simulink subsystem "Aerodyn"  (R2023b)
settings: Solver=VariableStepAuto  StartTime=0.0  StopTime=10.0  RelTol=1e-3
undefined symbols (not defined in the file): Aerodynamics
settings Model: Creator=NicolasS  LastModifiedBy=rouve
settings SolverCC: AlgebraicLoopSolver=TrustRegion
settings DebuggingCC: UnconnectedInputMsg=warning  UnconnectedOutputMsg=warning  UnconnectedLineMsg=warning
settings ModelReferenceCC: EnableRefExpFcnMdlSchedulingChecks=on
settings RTWCC: DLArmComputeVersion=19.05

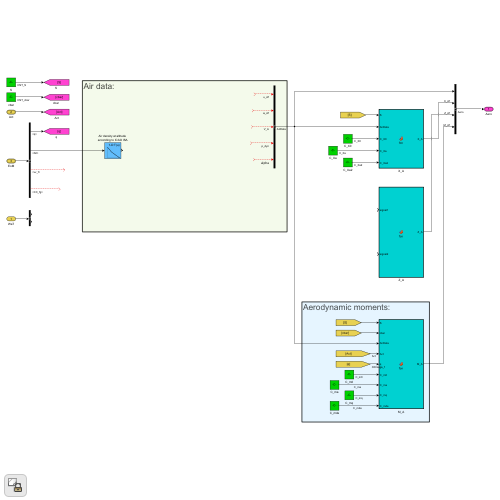
[thumbnail: Simulink's stored preview of the top-level diagram]
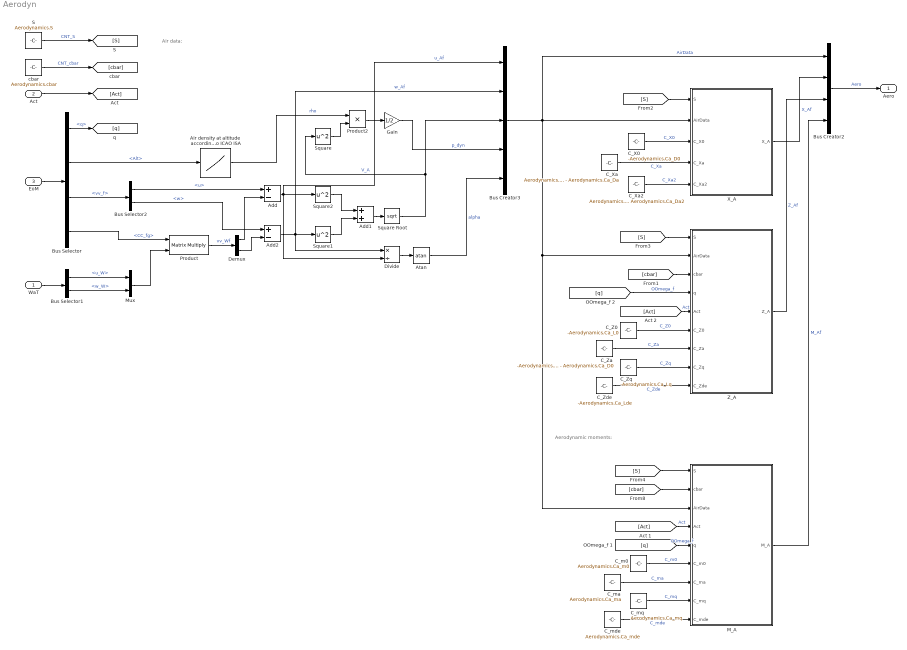
== system Aerodyn ==
  note: Aerodynamic moments:
  note: Air data:
  WaT : Inport  OutDataTypeStr=Bus: WaT
  Act : Inport  Port=2  OutDataTypeStr=Bus: Act
  EoM : Inport  Port=3  OutDataTypeStr=Bus: EoM
  Add : Sum  Inputs=+-
  Add1 : Sum
  Add2 : Sum  Inputs=+-
  Air density at altitude according to ICAO ISA : Lookup_n-D  NumberOfTableDimensions=1  BreakpointsForDimension1=Aerodynamics.LUT_Alt  Table=Aerodynamics.LUT_rho  ExtrapMethod=Clip  InternalRulePriority=Speed  RndMeth=Simplest
  Atan : Trigonometry  Operator=atan
  Bus Creator2 : BusCreator  Inputs=4  OutDataTypeStr=Bus: Aero
  Bus Creator3 : BusCreator  Inputs=5  OutDataTypeStr=Bus: AirData
  Bus Selector : BusSelector  OutputSignals=q,Alt,vv_f,CC.CC_fg
  Bus Selector1 : BusSelector  OutputSignals=u_W,w_W
  Bus Selector2 : BusSelector  OutputSignals=u,w
  C_X0 : Constant  Value=-Aerodynamics.Ca_D0  VectorParams1D=off  OutDataTypeStr=double  SampleTime=-1
  C_Xa : Constant  Value=Aerodynamics.Ca_L0 - Aerodynamics.Ca_Da  VectorParams1D=off  OutDataTypeStr=double  SampleTime=-1
  C_Xa2 : Constant  Value=Aerodynamics.Ca_La - Aerodynamics.Ca_Da2  VectorParams1D=off  OutDataTypeStr=double  SampleTime=-1
  C_Z0 : Constant  Value=-Aerodynamics.Ca_L0  VectorParams1D=off  OutDataTypeStr=double  SampleTime=-1
  C_Za : Constant  Value=-Aerodynamics.Ca_La - Aerodynamics.Ca_D0  VectorParams1D=off  OutDataTypeStr=double  SampleTime=-1
  C_Zde : Constant  Value=-Aerodynamics.Ca_Lde  VectorParams1D=off  OutDataTypeStr=double  SampleTime=-1
  C_Zq : Constant  Value=-Aerodynamics.Ca_Lq  VectorParams1D=off  OutDataTypeStr=double  SampleTime=-1
  C_m0 : Constant  Value=Aerodynamics.Ca_m0  VectorParams1D=off  OutDataTypeStr=double  SampleTime=-1
  C_ma : Constant  Value=Aerodynamics.Ca_ma  VectorParams1D=off  OutDataTypeStr=double  SampleTime=-1
  C_mde : Constant  Value=Aerodynamics.Ca_mde  VectorParams1D=off  OutDataTypeStr=double  SampleTime=-1
  C_mq : Constant  Value=Aerodynamics.Ca_mq  VectorParams1D=off  OutDataTypeStr=double  SampleTime=-1
  Demux : Demux  Outputs=2
  Divide : Product  Inputs=*/
  Gain : Gain  Gain=1/2
  M_A : MATLAB Function  TreatAsAtomicUnit=on
  Mux : Mux  Inputs=2
  Product : Product  Multiplication=Matrix(*)
  Product2 : Product
  S : Constant  Value=Aerodynamics.S  OutDataTypeStr=double  SampleTime=-1
  Square : Math  Operator=square
  Square Root : Sqrt
  Square1 : Math  Operator=square
  Square2 : Math  Operator=square
  X_A : MATLAB Function  TreatAsAtomicUnit=on
  Z_A : MATLAB Function  TreatAsAtomicUnit=on
  cbar : Constant  Value=Aerodynamics.cbar  OutDataTypeStr=double  SampleTime=-1
  Aero : Outport  OutDataTypeStr=Bus: Aero
  wires:
  C_m0/1 -> M_A/6(C_m0)  "C_m0"
  Bus Creator2/1 -> Aero/1  "Aero"
  C_mde/1 -> M_A/9(C_mde)  "C_mde"
  S/1 -> [S]  "CNT_S"
  C_Xa/1 -> X_A/4(C_Xa)  "C_Xa"
  Bus Creator3/1 -> X_A/2(AirData), Z_A/2(AirData), M_A/3(AirData), Bus Creator2/1  "AirData"
  EoM/1 -> Bus Selector/1
  M_A/1(M_A) -> Bus Creator2/4  "M_Af"
  Z_A/1(Z_A) -> Bus Creator2/3  "Z_Af"
  C_ma/1 -> M_A/7(C_ma)  "C_ma"
  C_mq/1 -> M_A/8(C_mq)  "C_mq"
  X_A/1(X_A) -> Bus Creator2/2  "X_Af"
  C_X0/1 -> X_A/3(C_X0)  "C_X0"
  [S] -> M_A/1(S)
  [q] -> M_A/5(q)  "OOmega_f"
  Gain/1 -> Bus Creator3/4  "p_dyn"
  [Act] -> M_A/4(Act)  "Act"
  [cbar] -> M_A/2(cbar)
  Bus Selector/2 -> Air density at altitude according to ICAO ISA/1  "<Alt>"
  C_Xa2/1 -> X_A/5(C_Xa2)  "C_Xa2"
  WaT/1 -> Bus Selector1/1
  cbar/1 -> [cbar]  "CNT_cbar"
  Bus Selector/1 -> [q]  "<q>"
  Act/1 -> [Act]
  Square Root/1 -> Bus Creator3/3, Square/1  "V_A"
  [S] -> X_A/1(S)
  Atan/1 -> Bus Creator3/5  "alpha"
  Bus Selector/3 -> Bus Selector2/1  "<vv_f>"
  Add2/1 -> Bus Creator3/2, Square1/1, Divide/1  "w_Af"
  Add/1 -> Bus Creator3/1, Square2/1, Divide/2  "u_Af"
  Bus Selector2/1 -> Add/1  "<u>"
  Bus Selector2/2 -> Add2/1  "<w>"
  Air density at altitude according to ICAO ISA/1 -> Product2/1  "rho"
  Square/1 -> Product2/2
  Product2/1 -> Gain/1
  Square2/1 -> Add1/1
  Square1/1 -> Add1/2
  Add1/1 -> Square Root/1
  Divide/1 -> Atan/1
  [Act] -> Z_A/5(Act)  "Act"
  C_Zde/1 -> Z_A/9(C_Zde)  "C_Zde"
  C_Zq/1 -> Z_A/8(C_Zq)  "C_Zq"
  C_Za/1 -> Z_A/7(C_Za)  "C_Za"
  C_Z0/1 -> Z_A/6(C_Z0)  "C_Z0"
  [cbar] -> Z_A/3(cbar)
  [q] -> Z_A/4(q)  "OOmega_f"
  Bus Selector1/2 -> Mux/2  "<w_W>"
  Bus Selector1/1 -> Mux/1  "<u_W>"
  Mux/1 -> Product/2
  Bus Selector/4 -> Product/1  "<CC_fg>"
  Product/1 -> Demux/1  "vv_Wf"
  Demux/2 -> Add2/2
  Demux/1 -> Add/2
  [S] -> Z_A/1(S)

== matlab function Aerodyn/Z_A ==
  data: S input; AirData input; cbar input; q input; Act input; Z_A output; C_Z0 input; C_Za input; C_Zq input; C_Zde input

%%%%%%%%%%%%%%%%%%%%%%
% Body-fixed Z force %
%%%%%%%%%%%%%%%%%%%%%%

function Z_A = fcn(S, AirData, cbar, q, Act, C_Z0, C_Za, C_Zq, C_Zde)

Z_A = AirData.p_dyn*S*(C_Z0 + C_Za*AirData.alpha + C_Zq*cbar/AirData.V_A *q + C_Zde*Act.de);

== matlab function Aerodyn/M_A ==
  data: S input; cbar input; AirData input Bus: AirData size=1; Act input; q input; C_m0 input; C_ma input; C_mq input; C_mde input; M_A output

%%%%%%%%%%%%%%%%%%%%%%%%%%%
% Body-fixed pitch moment %
%%%%%%%%%%%%%%%%%%%%%%%%%%%

function M_A = fcn(S,cbar,AirData,Act,q,C_m0,C_ma,C_mq,C_mde)

M_A = AirData.p_dyn*S*cbar*(C_m0 + C_ma*AirData.alpha + C_mq*q*cbar/AirData.V_A + C_mde*Act.de);

== matlab function Aerodyn/X_A ==
  data: S input; AirData input Bus: AirData size=1; C_X0 input; C_Xa input; C_Xa2 input; X_A output

%%%%%%%%%%%%%%%%%%%%%%
% Body-fixed X force %
%%%%%%%%%%%%%%%%%%%%%%

function X_A = fcn(S,AirData,C_X0,C_Xa,C_Xa2)

X_A = AirData.p_dyn*S*(C_X0 + C_Xa*AirData.alpha+C_Xa2*AirData.alpha^2);
